simulink model "imc_model"  (Simulink 8.5)
settings: Solver=ode4  StartTime=0.0  StopTime=10  FixedStep=1e-2  RelTol=1e-3
values from neighbouring files (symbols this model uses):
  Km = 1    [G_1.m]    (also in G_2.m; G_3.m; G_4.m; G_5.m)
  lambda = x(2)    [G_1.m]    (also in G_2.m; G_3.m; G_4.m; G_5.m)
  T = G3(1,i).den{1,1}(1)    [G_3.m]    (also in G_4.m = G4(1,i).den{1,1}(1); G_5.m = G5(1,i).den{1,1}(1); imc_skrypt.m = 1.1; main.m = G5(1,i).den{1,1}(1))
  Tm = x(1)    [G_1.m]    (also in G_2.m; G_3.m; G_4.m; G_5.m)
settings Model: Creator=student  LastModifiedBy=Adrian
settings DataIOCC: LimitDataPoints=off
settings DebuggingCC: SolverPrmCheckMsg=warning  FcnCallInpInsideContextMsg=EnableAllAsWarning
settings GRTTargetCC: CombineOutputUpdateFcns=on  GRTInterface=off

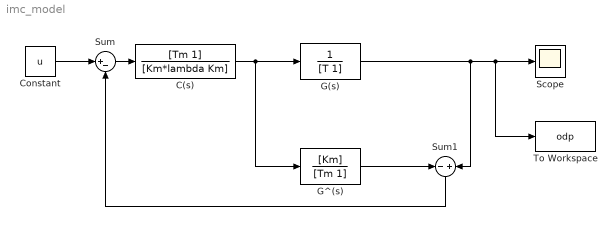
== system imc_model ==
  C(s) : TransferFcn  Numerator=[Tm 1]  Denominator=[Km*lambda Km]
  Constant : Constant  Value=u
  G(s) : TransferFcn  Denominator=[T 1]
  G^(s) : TransferFcn  Numerator=[Km]  Denominator=[Tm 1]
  Scope : Scope
  Sum : Sum  Inputs=|+-
  Sum1 : Sum  Inputs=-|+
  To Workspace : ToWorkspace  VariableName=odp  SaveFormat=Timeseries  SampleTime=-1
  wires:
  Sum/1 -> C(s)/1
  C(s)/1 -> G(s)/1, G^(s)/1
  G(s)/1 -> Sum1/2, Scope/1, To Workspace/1
  G^(s)/1 -> Sum1/1
  Sum1/1 -> Sum/2
  Constant/1 -> Sum/1
